simulink model "kart"  (R2025b)
settings: Solver=VariableStepAuto  StartTime=0.0  StopTime=10.0  RelTol=1e-3
libraries: instrumentseriallib x2, slrealtimeutilitieslib x1, nesl_utility x1
settings Model: Creator=Lenovo  LastModifiedBy=Lenovo

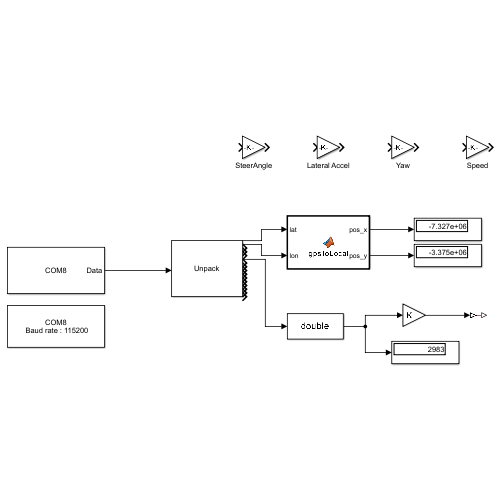
[thumbnail: Simulink's stored preview of the top-level diagram]
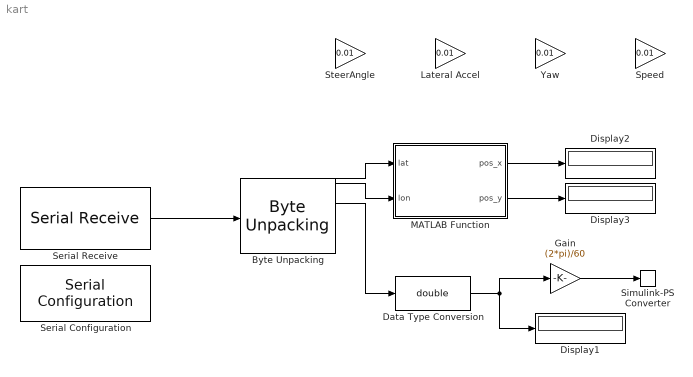
== system kart ==
  Byte Unpacking : slrealtimeutilitieslib/Byte Unpacking  MaskUnpackedDataTypes={'single', 'single', 'single', 'single', 'single', 'single', 'single', 'single', 'single', 'single', 'single', 'uint32', 'single', 'single', 'single', 'uint32'}  MaskUnpackedDataSizes={[1], [1], [1], [1], [1], [1], [1], [1], [1], [1], [1], [1], [1], [1], [1], [1]}  MaskAlignment=1
  Data Type Conversion : DataTypeConversion  OutDataTypeStr=double  SaturateOnIntegerOverflow=off  RndMeth=Floor  LockScale=on
  Display1 : Display
  Display2 : Display
  Display3 : Display
  Gain : Gain  Gain=(2*pi)/60
  Lateral Accel : Gain  Gain=0.01
  MATLAB Function : MATLAB Function  TreatAsAtomicUnit=on
  Serial Configuration : instrumentseriallib/Serial Configuration  Priority=-200000  PortSel=COM8  Port=COM8  ComPort=COM8  BaudRate=115200  DataBits=8  Parity=none  StopBits=1  ByteOrder=little-endian  FlowControl=none  Timeout=10  SimulateUsing=Interpreted execution  BlockInModel=on  aMode=1
  Serial Receive : instrumentseriallib/Serial Receive  Priority=1  PortSel=COM8  Port=COM8  ComPort=COM8  DataType=uint8  SaveDataType=uint8  ToggleHeader=off  Header=[170]  ToggleDataSize=on  DataSize=[64 1]  ToggleTerminator=off  Terminator=<none>  CustomTerminator=[]  InputFormat=Column major  EnableBlockingMode=on  ActionDataUnavailable=Output last received value  ActionWhenDataUnavailable=Output last received value  CustomValue=0  SampleTime=0.02  SimulateUsing=Interpreted execution  BlockInModel=on  aMode=1  LibraryInUse=instrumentlib
  Simulink-PS Converter : nesl_utility/Simulink-PS Converter  PhysicalDomain=network_engine_domain  SubClassName=ps_input  LeftPortType=input  RightPortType=output  PseudoPeriodic=off  Frequencies=[]  NoiseDistribution=none  NoiseParameters=[]  Unit=1  AffineConversion=off  FilteringAndDerivatives=provide  SimscapeFilterOrder=1  InputFilterTimeConstant=0.001  UdotUserProvided=0
  Speed : Gain  Gain=0.01
  SteerAngle : Gain  Gain=0.01
  Yaw : Gain  Gain=0.01
  wires:
  Serial Receive/1 -> Byte Unpacking/1
  MATLAB Function/1(pos_x) -> Display2/1
  Gain/1 -> Simulink-PS Converter/1
  Data Type Conversion/1 -> Display1/1, Gain/1
  Byte Unpacking/6 -> Data Type Conversion/1
  MATLAB Function/2(pos_y) -> Display3/1
  Byte Unpacking/1 -> MATLAB Function/1(lat)
  Byte Unpacking/2 -> MATLAB Function/2(lon)

== matlab function kart/MATLAB Function ==
  data: lat input; pos_x output; lon input; pos_y output
function [pos_x, pos_y] = gpsToLocal(lat, lon)
    % 1. Set the Reference Origin (Matches your Python Script)
    lat0 = 30.3527; 
    lon0 = 76.3608;
    
    % 2. Earth Radius (approximate)
    R = 6371000; % meters

    % 3. Calculate Differences in Degrees
    dLat = lat - lat0;
    dLon = lon - lon0;

    % 4. Convert to Meters (Simple Equirectangular Projection)
    % Latitude: 1 deg = ~111km
    pos_y = dLat * (pi/180) * R;
    
    % Longitude: 1 deg shrinks as you go north (cos(lat))
    pos_x = dLon * (pi/180) * R * cosd(lat0);
end
